simulink model "lev4coils"  (R2021b)
settings: Solver=ode3  StartTime=0.0  StopTime=15  FixedStep=1e-3  RelTol=1e-3
values from neighbouring files (symbols this model uses):
  g = s(1:n,n+1:n+nb)    [MagLev.m]    (also in MagLev4coils.m = 9.8)
  K1 = m*g/(2*b)    (= 5.40205233157e-05)    [MagLev4coils.m]
  K2 = K1    (= 5.40205233157e-05)    [MagLev4coils.m]
  K3 = K1    (= 5.40205233157e-05)    [MagLev4coils.m]
  K4 = K2    (= 5.40205233157e-05)    [MagLev4coils.m]
  l = 0.0567/2    (= 0.02835)    [MagLev4coils.m]
  L1 = L    (= 0.00388)    [MagLev4coils.m]
  L2 = L    (= 0.00388)    [MagLev4coils.m]
  m = 0.03    [MagLev.m]    (also in MagLev4coils.m = 0.01)
  R1 = R    (= 4)    [MagLev4coils.m]
  R2 = R    (= 4)    [MagLev4coils.m]
  x10x = x10x + i*0.004    [MagLev4coils.m]
  x10z = -0.03    [MagLev4coils.m]
settings Model: Creator=macbook_pro  LastModifiedBy=ik76

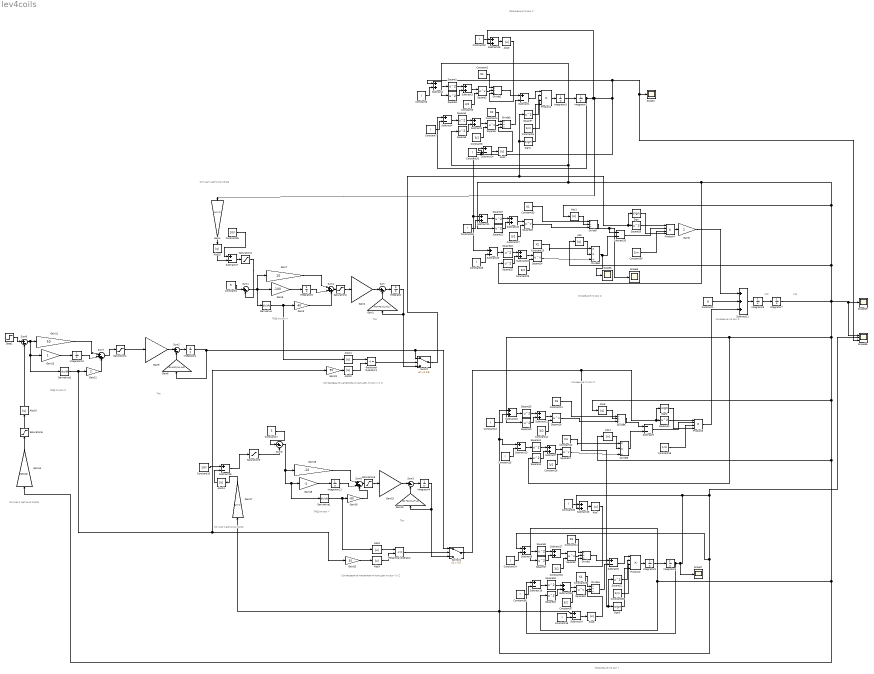
== system lev4coils ==
  note: Сигнал с датчика Холла
  note: Сигнал с датчика Холла
  note: Сигнал с датчика Холла
  note: Согласование напряжения катушек по оси Y и Z
  note: Согласование напряжения катушек по оси X и Z
  note: Ток
  note: Ток
  note: Ток
  note: ПИД по оси Y
  note: ПИД по оси Z
  note: ПИД по оси X
  note: Ускорение по оси Z
  note: Положение по оси X
  note: Положение по оси Y
  note: Ускорение по оси Z
  note: Ускорение по оси Z
  note: X1z
  note: X2z
  Abs{,1..13,15} (15 alike) : Abs
  Constant1 : Constant  Value=g
  Constant10 : Constant  Value=10/l
  Constant11 : Constant  Value=K3
  Constant12 : Constant  Value=K4
  Constant{5,7,13,15,19..20,24,26,28,31..32,36} (12 alike) : Constant  Value=l
  Constant{6,8,14,16,27,29,34,37} (8 alike) : Constant  Value=3/2
  Constant17 : Constant  Value=3
  Constant{9,18,30,38} (4 alike) : Constant  Value=1/m
  Constant2 : Constant  Value=K1
  Constant21 : Constant  Value=K3
  Constant23 : Constant  Value=K4
  Constant25 : Constant  Value=K2
  Constant3 : Constant  Value=5
  Constant33 : Constant  Value=K1
  Constant35 : Constant  Value=10/l
  Constant4 : Constant  Value=K2
  Derivative : Derivative
  Derivative1 : Derivative
  Derivative2 : Derivative
  Divide{1..4} (4 alike) : Product  Inputs=*/*
  Divide{5..8} (4 alike) : Product  Inputs=**/
  Gain1 : Gain  Gain=(R1+R2)/(L1+L2)
  Gain10 : Gain  Gain=(R1+R2)/(L1+L2)
  Gain11 : Gain  Gain=50
  Gain12 : Gain  Gain=2
  Gain13 : Gain
  Gain14 : Gain  Gain=(5/0.04)
  Gain15 : Gain  Gain=12/((L2+L1)*5)
  Gain16 : Gain  Gain=-60
  Gain17 : Gain  Gain=5/(l*2)
  Gain18 : Gain  Gain=-1
  Gain19 : Gain  Gain=-10
  Gain2 : Gain  Gain=12/((L2+L1)*5)
  Gain20 : Gain  Gain=55
  Gain21 : Gain  Gain=55
  Gain3 : Gain  Gain=-60
  Gain4 : Gain  Gain=5/(l*2)
  Gain5 : Gain
  Gain6 : Gain  Gain=-100
  Gain7 : Gain  Gain=10
  Gain8 : Gain  Gain=(R1+R2)/(L1+L2)
  Gain9 : Gain  Gain=12/((L2+L1)*5)
  Integrator{,1,3..4,6,8..11} (9 alike) : Integrator
  Integrator2 : Integrator  InitialCondition=x10x
  Integrator5 : Integrator  InitialCondition=1
  Integrator7 : Integrator  InitialCondition=x10z
  Product{1..4} (4 alike) : Product  Inputs=4
  Relational Operator : RelationalOperator  Operator=<=  OutDataTypeStr=boolean  RndMeth=Simplest
  Relational Operator1 : RelationalOperator  Operator=<=  OutDataTypeStr=boolean  RndMeth=Simplest
  Saturation1 : Saturate  UpperLimit=5  LowerLimit=0
  Saturation2 : Saturate  UpperLimit=5  LowerLimit=-5
  Saturation3 : Saturate  UpperLimit=5  LowerLimit=0
  Saturation4 : Saturate  UpperLimit=5  LowerLimit=-5
  Saturation5 : Saturate  UpperLimit=0  LowerLimit=-5
  Saturation6 : Saturate  UpperLimit=5  LowerLimit=-5
  Scope{1,3,5,7,19} (5 alike) : Scope
  Scope36 : Scope  NumInputPorts=3
  Sign{,1..3} (4 alike) : Signum
  Square{1,3..4,6..8,10..11,13..15,17..18,20..23,25..27} (20 alike) : Math  Operator=square  SaturateOnIntegerOverflow=on
  Square{2,5,9,12,16,19,24,28} (8 alike) : Math  Operator=pow  SaturateOnIntegerOverflow=on
  Step1 : Step  Time=0  After=3.5  SampleTime=0
  Subtract{1,4,6,13..14,18,23..24,27..28} (10 alike) : Sum  Inputs=+-
  Subtract{2..3,5,7..8,10,12,15,17,19,21..22,25..26} (14 alike) : Sum
  Subtract11 : Sum  Inputs=+++
  Subtract20 : Sum  Inputs=--
  Subtract9 : Sum  Inputs=--
  Sum{,1..3,5..6} (6 alike) : Sum  Inputs=|+-
  Sum4 : Sum  Inputs=|+++
  Sum7 : Sum  Inputs=|+++
  Sum8 : Sum  Inputs=|+++
  Switch : Switch  Threshold=0.5
  Switch1 : Switch  Criteria=u2 > Threshold  Threshold=0.5
  wires:
  Constant29/1 -> Square24/2
  Subtract23/1 -> Square23/1
  Sign1/1 -> Product1/4
  Integrator6/1 -> Integrator7/1
  Square7/1 -> Product1/2
  Derivative2/1 -> Gain12/1, Gain21/1, Gain20/1
  Subtract5/1 -> Square5/1
  Divide8/1 -> Scope3/1, Subtract20/2
  Step1/1 -> Sum6/1
  Subtract20/1 -> Product4/2
  Subtract3/1 -> Square2/1
  Subtract2/1 -> Square1/1
  Gain3/1 -> Sum4/3
  Square4/1 -> Subtract5/1
  Constant2/1 -> Divide2/1
  Subtract21/1 -> Square27/1
  Product1/1 -> Integrator3/1
  Constant1/1 -> Subtract11/2
  Square3/1 -> Subtract3/2
  Constant8/1 -> Square5/2
  Subtract27/1 -> Saturation1/1
  Constant4/1 -> Divide3/1
  Constant33/1 -> Divide7/1
  Divide7/1 -> Scope5/1, Subtract20/1
  Constant7/1 -> Subtract4/2
  Constant32/1 -> Subtract25/1
  Subtract24/1 -> Abs2/1
  Gain7/1 -> Sum4/1
  Subtract1/1 -> Product1/1
  Square6/1 -> Subtract5/2
  Square22/1 -> Subtract22/2
  Constant25/1 -> Divide8/1
  Subtract19/1 -> Square24/1
  Constant31/1 -> Subtract24/2
  Square27/1 -> Subtract22/1
  Integrator8/1 -> Sum4/2
  Square1/1 -> Subtract3/1
  Subtract22/1 -> Square28/1
  Constant30/1 -> Product4/3
  Abs2/1 -> Divide3/3
  Constant28/1 -> Subtract23/2
  Square25/1 -> Subtract19/2
  Constant26/1 -> Subtract21/2
  Integrator3/1 -> Integrator2/1
  Square28/1 -> Divide7/3
  Divide2/1 -> Subtract1/1
  Constant5/1 -> Subtract2/2
  Square26/1 -> Product4/1
  Constant27/1 -> Square28/2
  Square2/1 -> Divide2/2
  Subtract4/1 -> Square4/1
  Divide3/1 -> Subtract1/2
  Subtract25/1 -> Abs3/1
  Sum/1 -> Integrator/1
  Gain1/1 -> Sum/2
  Square5/1 -> Divide3/2
  Gain2/1 -> Sum/1
  Constant6/1 -> Square2/2
  Abs3/1 -> Divide2/3
  Saturation2/1 -> Gain2/1
  Subtract11/1 -> Integrator6/1
  Square24/1 -> Divide8/3
  Square23/1 -> Subtract19/1
  Switch/1 -> Square7/1, Sign1/1, Sign/1, Square26/1
  Constant9/1 -> Product1/3
  Integrator2/1 -> Subtract25/2, Scope36/3, Scope1/1, Subtract2/1, Subtract21/1, Subtract23/1, Subtract24/1, Gain4/1, Subtract4/1
  Sum1/1 -> Gain7/1, Gain6/1, Derivative/1
  Derivative/1 -> Abs11/1, Gain3/1
  Gain11/1 -> Sum7/1
  Sum7/1 -> Saturation4/1
  Integrator10/1 -> Sum7/2
  Gain13/1 -> Integrator10/1
  Saturation4/1 -> Gain9/1
  Sum4/1 -> Saturation2/1
  Gain6/1 -> Integrator8/1
  Saturation1/1 -> Sum1/2
  Constant3/1 -> Sum1/1
  Gain4/1 -> Abs15/1
  Abs/1 -> Divide8/2
  Abs1/1 -> Divide7/2
  Gain9/1 -> Sum2/1
  Sum2/1 -> Integrator1/1
  Gain8/1 -> Sum2/2
  Integrator/1 -> Switch/3, Gain1/1
  Sign/1 -> Product4/4
  Abs10/1 -> Sum6/2
  Product4/1 -> Gain5/1
  Gain15/1 -> Sum3/1
  Constant12/1 -> Divide6/1
  Square21/1 -> Product2/2
  Constant11/1 -> Divide1/1
  Constant34/1 -> Square9/2
  Integrator5/1 -> Scope7/1, Subtract15/2, Subtract10/1, Subtract13/1, Gain17/1, Subtract14/1, Subtract8/1, Scope36/2, Subtract18/1
  Subtract10/1 -> Square15/1
  Subtract6/1 -> Product2/1
  Constant21/1 -> Divide5/1
  Divide4/1 -> Subtract6/2
  Product2/1 -> Integrator9/1
  Constant16/1 -> Square12/2
  Subtract28/1 -> Saturation3/1
  Subtract13/1 -> Square11/1
  Square16/1 -> Divide5/3
  Square17/1 -> Subtract17/2
  Constant20/1 -> Subtract15/1
  Subtract17/1 -> Square9/1
  Sum3/1 -> Integrator4/1
  Square9/1 -> Divide1/2
  Subtract14/1 -> Abs6/1
  Square18/1 -> Subtract26/1
  Subtract7/1 -> Square12/1
  Constant37/1 -> Square19/2
  Constant19/1 -> Subtract14/2
  Divide1/1 -> Subtract6/1
  Integrator7/1 -> Square13/1, Square10/1, Abs5/1, Abs4/1, Square17/1, Square20/1, Gain14/1, Abs/1, Abs1/1, Square25/1, Square3/1, Square6/1, Square22/1, Scope36/1, Scope19/1
  Gain10/1 -> Sum3/2
  Square20/1 -> Subtract26/2
  Square15/1 -> Subtract12/1
  Integrator11/1 -> Sum8/2
  Subtract12/1 -> Square16/1
  Constant36/1 -> Subtract18/2
  Subtract26/1 -> Square19/1
  Square13/1 -> Subtract7/2
  Divide6/1 -> Subtract9/2
  Integrator9/1 -> Integrator5/1
  Constant18/1 -> Product3/3
  Subtract8/1 -> Square8/1
  Constant14/1 -> Square16/2
  Subtract18/1 -> Square18/1
  Subtract15/1 -> Abs7/1
  Square10/1 -> Subtract12/2
  Square19/1 -> Divide4/2
  Constant13/1 -> Subtract10/2
  Saturation6/1 -> Gain15/1
  Square8/1 -> Subtract17/1
  Gain17/1 -> Abs13/1
  Square14/1 -> Product3/1
  Square12/1 -> Divide6/3
  Divide5/1 -> Subtract9/1
  Square11/1 -> Subtract7/1
  Constant15/1 -> Subtract13/2
  Subtract9/1 -> Product3/2
  Constant38/1 -> Product2/3
  Constant23/1 -> Divide4/1
  Gain19/1 -> Sum8/1
  Sum5/1 -> Derivative1/1, Gain18/1, Gain19/1
  Sum8/1 -> Saturation6/1
  Constant24/1 -> Subtract8/2
  Saturation3/1 -> Sum5/2
  Constant17/1 -> Sum5/1
  Abs7/1 -> Divide1/3
  Sign3/1 -> Product2/4
  Abs6/1 -> Divide4/3
  Switch1/1 -> Square21/1, Sign3/1, Sign2/1, Square14/1
  Integrator4/1 -> Switch1/3, Gain10/1
  Abs5/1 -> Divide5/2
  Abs4/1 -> Divide6/2
  Sign2/1 -> Product3/4
  Product3/1 -> Subtract11/3
  Gain14/1 -> Saturation5/1
  Saturation5/1 -> Abs10/1
  Gain5/1 -> Subtract11/1
  Abs8/1 -> Relational Operator/1
  Abs9/1 -> Relational Operator/2
  Relational Operator/1 -> Switch1/2
  Sum6/1 -> Derivative2/1, Gain13/1, Gain11/1
  Gain12/1 -> Sum7/3
  Gain16/1 -> Sum8/3
  Gain18/1 -> Integrator11/1
  Derivative1/1 -> Abs8/1, Gain16/1
  Abs12/1 -> Relational Operator1/2
  Abs11/1 -> Relational Operator1/1
  Integrator1/1 -> Switch1/1, Switch/1, Gain8/1
  Relational Operator1/1 -> Switch/2
  Gain20/1 -> Abs9/1
  Gain21/1 -> Abs12/1
  Abs13/1 -> Subtract28/2
  Constant10/1 -> Subtract28/1
  Constant35/1 -> Subtract27/1
  Abs15/1 -> Subtract27/2
